simulink model "ZadacaII49"  (R2021a)
settings: Solver=VariableStepAuto  StartTime=0.0  StopTime=10.0  RelTol=1e-3
settings Model: Creator=stojo  LastModifiedBy=stojo

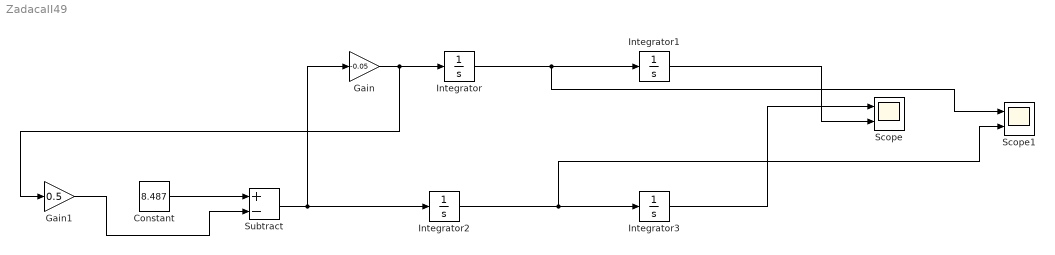
== system ZadacaII49 ==
  Constant : Constant  Value=8.487
  Gain : Gain  Gain=-0.05
  Gain1 : Gain  Gain=0.5
  Integrator{,1..3} (4 alike) : Integrator
  Scope : Scope  NumInputPorts=2
  Scope1 : Scope  NumInputPorts=2
  Subtract : Sum  Inputs=+-
  wires:
  Integrator2/1 -> Scope1/2, Integrator3/1
  Integrator/1 -> Scope1/1, Integrator1/1
  Subtract/1 -> Gain/1, Integrator2/1
  Gain/1 -> Gain1/1, Integrator/1
  Constant/1 -> Subtract/1
  Gain1/1 -> Subtract/2
  Integrator1/1 -> Scope/2
  Integrator3/1 -> Scope/1
